simulink model "AER821_Gimbal_part-1_rxn_wheel"  (R2025a)
settings: Solver=VariableStepAuto  StartTime=0.0  StopTime=10.0  RelTol=1e-3
libraries: simulink_extras x2
settings Model: Creator=bosco  LastModifiedBy=bosco

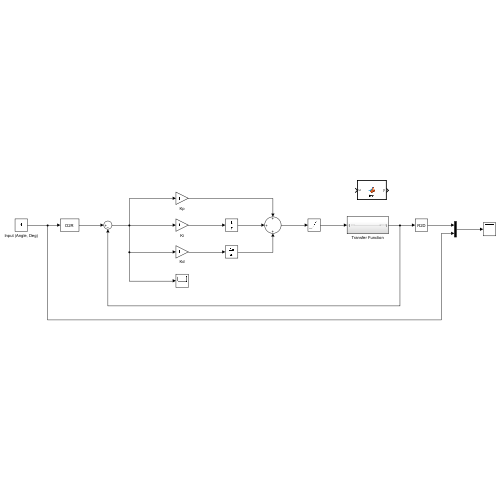
[thumbnail: Simulink's stored preview of the top-level diagram]
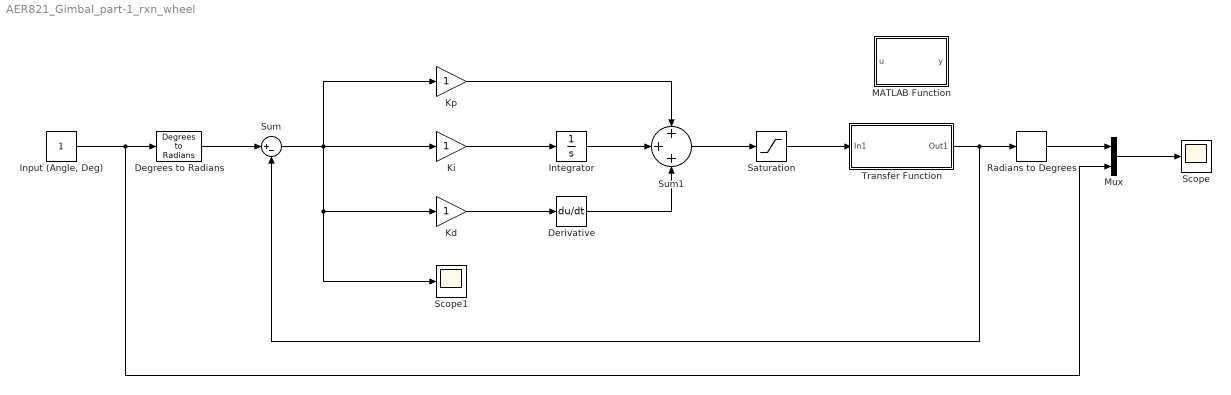
== system AER821_Gimbal_part-1_rxn_wheel ==
  Degrees to Radians : simulink_extras/Transformations/Degrees to Radians
  Derivative : Derivative
  "Input (Angle, Deg)" : Constant
  Integrator : Integrator
  Kd : Gain
  Ki : Gain
  Kp : Gain
  MATLAB Function : MATLAB Function  TreatAsAtomicUnit=on
  Mux : Mux  Inputs=2
  Radians to Degrees : simulink_extras/Transformations/Radians to Degrees
  Saturation : Saturate
  Scope : Scope
  Scope1 : Scope
  Sum : Sum  Inputs=|+-
  Sum1 : Sum  Inputs=+++
  Transfer Function : Subsystem
  wires:
  "Input (Angle, Deg)"/1 -> Mux/2, Degrees to Radians/1
  Degrees to Radians/1 -> Sum/1
  Ki/1 -> Integrator/1
  Kd/1 -> Derivative/1
  Integrator/1 -> Sum1/2
  Derivative/1 -> Sum1/3
  Kp/1 -> Sum1/1
  Sum1/1 -> Saturation/1
  Sum/1 -> Scope1/1, Kd/1, Kp/1, Ki/1
  Saturation/1 -> Transfer Function/1(In1)
  Transfer Function/1(Out1) -> Sum/2, Radians to Degrees/1
  Mux/1 -> Scope/1
  Radians to Degrees/1 -> Mux/1

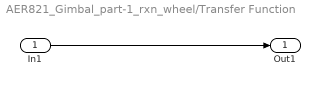
== system AER821_Gimbal_part-1_rxn_wheel/Transfer Function ==
  In1 : Inport
  Out1 : Outport
  wires:
  In1/1 -> Out1/1

== matlab function AER821_Gimbal_part-1_rxn_wheel/MATLAB Function ==
  data: u input; y output
function y = fcn(u)

y = u;
